simulink library "tpm"  (R2021b)
settings: Solver=VariableStepAuto  StartTime=0.0  StopTime=10.0  RelTol=1e-3
undefined symbols (not defined in the file or in its folder): ENUM_AN_LF, ENUM_AN_LR, ENUM_AN_RF, ENUM_AN_RR, ENUM_POWERSTA_OFF, ENUM_POWERSTA_OFFA, ENUM_POWERSTA_OFFC, ENUM_POWERSTA_ON, ENUM_POWERSTA_READY, ENUM_POWERSTA_STANDBY, ENUM_PWRSTASW_OFF, ENUM_PWRSTASW_OFFA, ENUM_PWRSTASW_OFFCHVCHRG, ENUM_PWRSTASW_STANDBY, ENUM_TPMSSNESORIDREGSTA_START, FALSE, KTPM_DataInVehSpdThreshold_kph, KTPM_Delay_raw8, KTPM_DiagLearn_flg, KTPM_TPMSModelVersion_raw, KTPM_TPMSModelVersionInit_raw, KTPM_WhlRotDir_enum_ovrdflg, KTPM_WhlRotDir_enum_ovrdval, TRUE, ZERO_FLOAT, ZERO_INT
libraries: simulink x58, $bdroot x27, hcu_lib x24
(part 6 of 9)

== system tpm/TPM/TPMS/TPMS/Learn/AutoLocation/IDIdentify/Subsystem3 ==
  VINP_DATAin_flg : Inport
  VINP_TPMSResButt_flg : Inport  Port=2
  VINP_IDin_raw32 : Inport  Port=3
  VTPM_LFWP_raw16 : Inport  Port=4
  VTPM_RFWP_raw16 : Inport  Port=5
  VTPM_LRWP_raw16 : Inport  Port=6
  VTPM_RRWP_raw16 : Inport  Port=7
  VPMM_PowerSta_enum : Inport  Port=8
  VINP_VehSpeed_kph : Inport  Port=9
  VINP_S4ID_raw : Inport  Port=10
  VTPM_TPMSmanualDone_flg : Inport  Port=11
  Add : Sum
  Chart : Stateflow chart  TreatAsAtomicUnit=on
      settings: PortSchema="{\"entries\":[{\"content\":{\"sides\":[{\"content\":{\"connectorIds\":[\"In1\",\"In2\",\"In3\",\"In5\",\"In7\",\"In4\",\"In6\"]},\"type\":\"ConnectorPlacement.EquallySpacedRectSide\",\"uuid\":\"84bbdee3-6a13-4113-bc08-a0b87ba22909\"},{\"content\":{\"connectorIds\":[\"Out5\",\"Out1\",\"Out4\",\"Out2\",\"Out3\"],\"side\":\"RIGHT\"},\"type\":\"ConnectorPlacement.EquallySpacedRectSide\",\"uuid\":\"b8796851-ab69-429f-9540-9571864c98e0\"},{\"content\":{\"connectorIds\":[],\"side\":\"TOP\"},\"type\":\"ConnectorPlacement.EquallySpacedRectSide\",\"uuid\":\"52bdbec4-409e-4a9a-a4bb-373a9525aed8\"}]},\"type\":\"ConnectorPlacement.EquallySpacedConnector\",\"uuid\":\"6e0a7370-38f8-4d4e-a3e7-eb2ef4c24b0f\"}],\"packageUris\":[\"http://schema.mathworks.com/mf0/Connector/R2020b\"],\"version\":\"1.0\"}"
  Chart1 : Stateflow chart  TreatAsAtomicUnit=on
      settings: PortSchema="{\"entries\":[{\"content\":{\"sides\":[{\"content\":{\"connectorIds\":[\"In2\",\"In1\",\"In3\",\"In4\",\"In5\",\"In6\",\"In7\",\"In8\"]},\"type\":\"ConnectorPlacement.EquallySpacedRectSide\",\"uuid\":\"0106c0c7-b0dd-4985-8477-027279f2cfbe\"},{\"content\":{\"connectorIds\":[\"Out1\",\"Out2\",\"Out3\",\"Out4\",\"Out5\"],\"side\":\"RIGHT\"},\"type\":\"ConnectorPlacement.EquallySpacedRectSide\",\"uuid\":\"38b36b5e-8790-43f5-89a8-de723ff40088\"},{\"content\":{\"connectorIds\":[],\"side\":\"TOP\"},\"type\":\"ConnectorPlacement.EquallySpacedRectSide\",\"uuid\":\"aa12a430-979d-4bba-b5af-88414204d80d\"}]},\"type\":\"ConnectorPlacement.EquallySpacedConnector\",\"uuid\":\"9f6249c4-6459-404e-8830-3ea500254943\"}],\"packageUris\":[\"http://schema.mathworks.com/mf0/Connector/R2020b\"],\"version\":\"1.0\"}"
  Constant : Constant  Value=ZERO_INT
  Constant18 : Constant  Value=0
  Constant5 : Constant  Value=KTPM_DataInVehSpdThreshold_kph  OutDataTypeStr=single
  Data Type Conversion10 : DataTypeConversion  OutDataTypeStr=uint32
  Detect Increase : simulink/Logic and Bit Operations/Detect Increase  vinit=0.0  OutDataTypeStr=boolean
  Enabled Subsystem1 : Subsystem  TreatAsAtomicUnit=on
  Enabled Subsystem2 : Subsystem  TreatAsAtomicUnit=on
  Enabled Subsystem3 : Subsystem  TreatAsAtomicUnit=on
  Enabled Subsystem5 : Subsystem  TreatAsAtomicUnit=on
  Logical Operator : Logic  Operator=OR  AllPortsSameDT=off  OutDataTypeStr=boolean
  NOT : Logic  Operator=NOT  IconShape=distinctive  AllPortsSameDT=off  OutDataTypeStr=boolean
  Relational Operator : RelationalOperator  Operator=~=  OutDataTypeStr=boolean  RndMeth=Simplest
  Switch5 : Switch  Criteria=u2 > Threshold
  Unit Delay1 : UnitDelay  SampleTime=-1  HasFrameUpgradeWarning=on
  IDOut : Outport
  VTPM_S4IDLock_flg : Outport  Port=2
  Used : Outport  Port=3
  VTPM_LFS4_cnt : Outport  Port=4
  VTPM_RFS4_cnt : Outport  Port=5
  VTPM_LRS4_cnt : Outport  Port=6
  VTPM_RRS4_cnt : Outport  Port=7
  C : Outport  Port=8
  GS4 : Outport  Port=9
  VTPM_S4timeout_flg : Outport  Port=10
  wires:
  VPMM_PowerSta_enum/1 -> Chart/2(VPMM_PowerSta_enum)
  Constant18/1 -> Switch5/1
  [VINP_TPMSResButt_flg] -> Switch5/2
  Data Type Conversion10/1 -> Add/1
  Unit Delay1/1 -> Add/2
  Switch5/1 -> [VTPM_GS4_cnt], Unit Delay1/1  "VTPM_GS4_cnt"
  Add/1 -> Switch5/3
  [C] -> Detect Increase/1
  Enabled Subsystem3/1(S) -> VTPM_RRS4_cnt/1
  Enabled Subsystem2/1(S) -> VTPM_LRS4_cnt/1
  Enabled Subsystem1/1(S) -> VTPM_RFS4_cnt/1
  [C] -> C/1
  Enabled Subsystem5/1(S) -> VTPM_LFS4_cnt/1
  Chart/3(RRM) -> Enabled Subsystem3/2(LFM1)
  [Cal] -> Enabled Subsystem3/Enable
  [C] -> Enabled Subsystem3/1(C)
  [C] -> Enabled Subsystem2/1(C)
  [Cal] -> Enabled Subsystem2/Enable
  Chart/2(LRM) -> Enabled Subsystem2/2(LFM1)
  Chart/4(RFM) -> Enabled Subsystem1/2(LFM1)
  [Cal] -> Enabled Subsystem1/Enable
  [C] -> Enabled Subsystem1/1(C)
  [C] -> Enabled Subsystem5/1(C)
  VINP_IDin_raw32/1 -> [VINP_IDin_raw32]
  VINP_TPMSResButt_flg/1 -> [VINP_TPMSResButt_flg]
  [VINP_TPMSResButt_flg] -> Logical Operator/2
  VTPM_RFWP_raw16/1 -> Chart/7(RF_PC)
  VTPM_RRWP_raw16/1 -> Chart/6(RR_PC)
  VTPM_LFWP_raw16/1 -> Chart/5(LF_PC)
  VTPM_LRWP_raw16/1 -> Chart/4(LR_PC)
  [G] -> Chart/3(GS)
  [VINP_TPMSResButt_flg] -> Chart1/2(VINP_TPMSResButt_flg)
  [VTPM_S4IDLock_flg] -> VTPM_S4IDLock_flg/1
  [VINP_IDin_raw32] -> Chart1/1(VINP_IDin_raw32)
  VINP_DATAin_flg/1 -> Chart1/3(VINP_DATAin_flg)
  Chart1/4(IDout) -> IDOut/1
  Chart1/1(G) -> GS4/1, [G], Data Type Conversion10/1
  Chart1/3(VTPM_S4IDLock_flg) -> [VTPM_S4IDLock_flg]
  Chart1/2(Used) -> [Used]
  [Used] -> Used/1
  Logical Operator/1 -> Chart/1(VINP_TPMSResButt_flg)
  [Used] -> NOT/1
  NOT/1 -> Logical Operator/1
  Chart/5(C) -> [C]
  [Cal] -> Enabled Subsystem5/Enable
  Chart/1(LFM) -> Enabled Subsystem5/2(LFM1)
  Detect Increase/1 -> [Cal]
  VINP_S4ID_raw/1 -> Relational Operator/1, [VINP_S4ID_raw]
  Constant/1 -> Relational Operator/2
  Relational Operator/1 -> [VTPM_FlashIDlock_flg]
  [VTPM_FlashIDlock_flg] -> Chart1/4(VTPM_FlashIDlock_flg)
  [VINP_S4ID_raw] -> Chart1/5(VINP_S4ID_raw)
  VINP_VehSpeed_kph/1 -> Chart1/6(VINP_VehSpeed_kph)
  Chart1/5(VTPM_S4timeout_flg) -> VTPM_S4timeout_flg/1
  VTPM_TPMSmanualDone_flg/1 -> Chart1/7(VTPM_TPMSmanualDone_flg)
  Constant5/1 -> Chart1/8(KTPM_DataInVehSpdThreshold_kph)

== system tpm/TPM/TPMS/TPMS/Learn/AutoLocation/IDIdentify/Subsystem7 ==
  VINP_DATAin_flg : Inport
  VINP_TPMSResButt_flg : Inport  Port=2
  VINP_IDin_raw32 : Inport  Port=3
  VTPM_LFWP_raw16 : Inport  Port=4
  VTPM_RFWP_raw16 : Inport  Port=5
  VTPM_LRWP_raw16 : Inport  Port=6
  VTPM_RRWP_raw16 : Inport  Port=7
  VPMM_PowerSta_enum : Inport  Port=8
  VINP_VehSpeed_kph : Inport  Port=9
  VINP_S1ID_raw : Inport  Port=10
  VTPM_TPMSmanualDone_flg : Inport  Port=11
  Add : Sum
  Chart : Stateflow chart  TreatAsAtomicUnit=on
      settings: PortSchema="{\"entries\":[{\"content\":{\"sides\":[{\"content\":{\"connectorIds\":[\"In1\",\"In2\",\"In3\",\"In5\",\"In7\",\"In4\",\"In6\"]},\"type\":\"ConnectorPlacement.EquallySpacedRectSide\",\"uuid\":\"84bbdee3-6a13-4113-bc08-a0b87ba22909\"},{\"content\":{\"connectorIds\":[\"Out5\",\"Out1\",\"Out4\",\"Out2\",\"Out3\"],\"side\":\"RIGHT\"},\"type\":\"ConnectorPlacement.EquallySpacedRectSide\",\"uuid\":\"b8796851-ab69-429f-9540-9571864c98e0\"},{\"content\":{\"connectorIds\":[],\"side\":\"TOP\"},\"type\":\"ConnectorPlacement.EquallySpacedRectSide\",\"uuid\":\"52bdbec4-409e-4a9a-a4bb-373a9525aed8\"}]},\"type\":\"ConnectorPlacement.EquallySpacedConnector\",\"uuid\":\"6e0a7370-38f8-4d4e-a3e7-eb2ef4c24b0f\"}],\"packageUris\":[\"http://schema.mathworks.com/mf0/Connector/R2020b\"],\"version\":\"1.0\"}"
  Chart1 : Stateflow chart  TreatAsAtomicUnit=on
      settings: PortSchema="{\"entries\":[{\"content\":{\"sides\":[{\"content\":{\"connectorIds\":[\"In2\",\"In1\",\"In3\",\"In4\",\"In5\",\"In6\",\"In7\",\"In8\"]},\"type\":\"ConnectorPlacement.EquallySpacedRectSide\",\"uuid\":\"0106c0c7-b0dd-4985-8477-027279f2cfbe\"},{\"content\":{\"connectorIds\":[\"Out1\",\"Out2\",\"Out3\",\"Out4\",\"Out5\"],\"side\":\"RIGHT\"},\"type\":\"ConnectorPlacement.EquallySpacedRectSide\",\"uuid\":\"38b36b5e-8790-43f5-89a8-de723ff40088\"},{\"content\":{\"connectorIds\":[],\"side\":\"TOP\"},\"type\":\"ConnectorPlacement.EquallySpacedRectSide\",\"uuid\":\"aa12a430-979d-4bba-b5af-88414204d80d\"}]},\"type\":\"ConnectorPlacement.EquallySpacedConnector\",\"uuid\":\"9f6249c4-6459-404e-8830-3ea500254943\"}],\"packageUris\":[\"http://schema.mathworks.com/mf0/Connector/R2020b\"],\"version\":\"1.0\"}"
  Constant : Constant  Value=ZERO_INT
  Constant18 : Constant  Value=0
  Constant5 : Constant  Value=KTPM_DataInVehSpdThreshold_kph  OutDataTypeStr=single
  Data Type Conversion10 : DataTypeConversion  OutDataTypeStr=uint32
  Detect Increase : simulink/Logic and Bit Operations/Detect Increase  vinit=0.0  OutDataTypeStr=boolean
  Enabled Subsystem1 : Subsystem  TreatAsAtomicUnit=on
  Enabled Subsystem2 : Subsystem  TreatAsAtomicUnit=on
  Enabled Subsystem3 : Subsystem  TreatAsAtomicUnit=on
  Enabled Subsystem5 : Subsystem  TreatAsAtomicUnit=on
  Logical Operator : Logic  Operator=OR  AllPortsSameDT=off  OutDataTypeStr=boolean
  NOT : Logic  Operator=NOT  IconShape=distinctive  AllPortsSameDT=off  OutDataTypeStr=boolean
  Relational Operator : RelationalOperator  Operator=~=  OutDataTypeStr=boolean  RndMeth=Simplest
  Switch5 : Switch  Criteria=u2 > Threshold
  Unit Delay1 : UnitDelay  SampleTime=-1  HasFrameUpgradeWarning=on
  IDOut : Outport
  VTPM_S1IDLock_flg : Outport  Port=2
  Used : Outport  Port=3
  VTPM_LFS1_cnt : Outport  Port=4
  VTPM_RFS1_cnt : Outport  Port=5
  VTPM_LRS1_cnt : Outport  Port=6
  VTPM_RRS1_cnt : Outport  Port=7
  C : Outport  Port=8
  GS1 : Outport  Port=9
  VTPM_S1timeout_flg : Outport  Port=10
  wires:
  Detect Increase/1 -> [Cal]
  Chart/1(LFM) -> Enabled Subsystem5/2(LFM1)
  [Cal] -> Enabled Subsystem5/Enable
  Chart/5(C) -> [C]
  NOT/1 -> Logical Operator/1
  [Used] -> NOT/1
  Logical Operator/1 -> Chart/1(VINP_TPMSResButt_flg)
  [Used] -> Used/1
  Chart1/2(Used) -> [Used]
  Chart1/3(VTPM_S1IDLock_flg) -> [VTPM_S1IDLock_flg]
  Chart1/1(G) -> Data Type Conversion10/1, GS1/1, [G]
  Chart1/4(IDout) -> IDOut/1
  VINP_DATAin_flg/1 -> Chart1/3(VINP_DATAin_flg)
  [VINP_IDin_raw32] -> Chart1/1(VINP_IDin_raw32)
  [VTPM_S1IDLock_flg] -> VTPM_S1IDLock_flg/1
  [VINP_TPMSResButt_flg] -> Chart1/2(VINP_TPMSResButt_flg)
  [G] -> Chart/3(GS)
  VTPM_LRWP_raw16/1 -> Chart/4(LR_PC)
  VTPM_LFWP_raw16/1 -> Chart/5(LF_PC)
  VTPM_RRWP_raw16/1 -> Chart/6(RR_PC)
  VTPM_RFWP_raw16/1 -> Chart/7(RF_PC)
  [VINP_TPMSResButt_flg] -> Logical Operator/2
  VINP_TPMSResButt_flg/1 -> [VINP_TPMSResButt_flg]
  VINP_IDin_raw32/1 -> [VINP_IDin_raw32]
  [C] -> Enabled Subsystem5/1(C)
  [C] -> Enabled Subsystem1/1(C)
  [Cal] -> Enabled Subsystem1/Enable
  Chart/4(RFM) -> Enabled Subsystem1/2(LFM1)
  Chart/2(LRM) -> Enabled Subsystem2/2(LFM1)
  [Cal] -> Enabled Subsystem2/Enable
  [C] -> Enabled Subsystem2/1(C)
  [C] -> Enabled Subsystem3/1(C)
  [Cal] -> Enabled Subsystem3/Enable
  Chart/3(RRM) -> Enabled Subsystem3/2(LFM1)
  Enabled Subsystem5/1(S) -> VTPM_LFS1_cnt/1
  [C] -> C/1
  Enabled Subsystem1/1(S) -> VTPM_RFS1_cnt/1
  Enabled Subsystem2/1(S) -> VTPM_LRS1_cnt/1
  Enabled Subsystem3/1(S) -> VTPM_RRS1_cnt/1
  [C] -> Detect Increase/1
  Add/1 -> Switch5/3
  Switch5/1 -> Unit Delay1/1, [VTPM_GS1_cnt]  "VTPM_GS1_cnt"
  Unit Delay1/1 -> Add/2
  Data Type Conversion10/1 -> Add/1
  [VINP_TPMSResButt_flg] -> Switch5/2
  Constant18/1 -> Switch5/1
  VPMM_PowerSta_enum/1 -> Chart/2(VPMM_PowerSta_enum)
  VINP_VehSpeed_kph/1 -> Chart1/6(VINP_VehSpeed_kph)
  VINP_S1ID_raw/1 -> [VINP_S1ID_raw], Relational Operator/1
  Relational Operator/1 -> [VTPM_FlashIDlock_flg]
  Constant/1 -> Relational Operator/2
  [VTPM_FlashIDlock_flg] -> Chart1/4(VTPM_FlashIDlock_flg)
  [VINP_S1ID_raw] -> Chart1/5(VINP_S1ID_raw)
  Chart1/5(VTPM_S1timeout_flg) -> VTPM_S1timeout_flg/1
  VTPM_TPMSmanualDone_flg/1 -> Chart1/7(VTPM_TPMSmanualDone_flg)
  Constant5/1 -> Chart1/8(KTPM_DataInVehSpdThreshold_kph)

== system tpm/TPM/TPMS/TPMS/Learn/AutoLocation/IDIdentify/unlearnsensorfail  ==
  VTPM_ALLFIN_flg : Inport
  VINP_VehSpeed_kph : Inport  Port=2
  VTPM_IDLOCK_flg : Inport  Port=3
  GS1 : Inport  Port=4
  GS2 : Inport  Port=5
  GS3 : Inport  Port=6
  GS4 : Inport  Port=7
  VINP_TPMSResButt_flg : Inport  Port=8
  VINP_FlashunlearnSfali_flg : Inport  Port=9
  VINP_ChkStorge_flg : Inport  Port=10
  VINP_TPMSStorge_flg : Inport  Port=11
  VTPM_TPMSmanualDone_flg : Inport  Port=12
  Chart : Stateflow chart  TreatAsAtomicUnit=on
      settings: PortSchema="{\"entries\":[{\"content\":{\"sides\":[{\"content\":{\"connectorIds\":[\"In1\",\"In2\",\"In3\",\"In7\",\"In4\",\"In5\",\"In6\",\"In8\",\"In9\",\"In10\",\"In11\",\"In12\"]},\"type\":\"ConnectorPlacement.EquallySpacedRectSide\",\"uuid\":\"6d6ad79b-53cb-4fcc-b2ed-afc1b708014e\"},{\"content\":{\"connectorIds\":[\"Out1\",\"Out2\"],\"side\":\"RIGHT\"},\"type\":\"ConnectorPlacement.EquallySpacedRectSide\",\"uuid\":\"e1142f2b-ba58-4cb3-ba57-f7dfdeb40e8a\"},{\"content\":{\"connectorIds\":[],\"side\":\"TOP\"},\"type\":\"ConnectorPlacement.EquallySpacedRectSide\",\"uuid\":\"d6c2cba7-0cc1-4e16-8027-e1abdfd1a8ea\"}]},\"type\":\"ConnectorPlacement.EquallySpacedConnector\",\"uuid\":\"635c654b-7cdc-40ae-8580-2307d04d13e7\"}],\"packageUris\":[\"http://schema.mathworks.com/mf0/Connector/R2020b\"],\"version\":\"1.0\"}"
  Detect Increase4 : simulink/Logic and Bit Operations/Detect Increase  vinit=0.0  OutDataTypeStr=boolean
  SR_Latch : hcu_lib/Basic_Blocks/SR_Latch
  SR_Latch1 : hcu_lib/Basic_Blocks/SR_Latch
  VTPM_unlearnSfali_flg : Outport
  VTPM_unlearnSfailvalid_enum : Outport  Port=2
  VTPM_unlockpopup_flg : Outport  Port=3
  wires:
  Chart/1(VTPM_unlearnSfali_flg) -> VTPM_unlearnSfali_flg/1, [VTPM_unlearnSfali_flg]
  GS1/1 -> Chart/7(VTPM_GS1_flg)
  GS4/1 -> Chart/6(VTPM_GS4_flg)
  GS3/1 -> Chart/5(VTPM_GS3_flg)
  GS2/1 -> Chart/4(VTPM_GS2_flg)
  VTPM_IDLOCK_flg/1 -> Chart/3(VTPM_IDLOCK_flg)
  VINP_VehSpeed_kph/1 -> Chart/2(VINP_VehSpeed_kph)
  VTPM_ALLFIN_flg/1 -> Chart/1(VTPM_ALLFIN_flg)
  VINP_FlashunlearnSfali_flg/1 -> Chart/9(VINP_FlashunlearnSfali_flg)
  VINP_ChkStorge_flg/1 -> Chart/10(VINP_ChkStorge_flg)
  VINP_TPMSStorge_flg/1 -> Chart/11(VINP_TPMSStorge_flg)
  SR_Latch/1 -> VTPM_unlearnSfailvalid_enum/1
  Detect Increase4/1 -> SR_Latch/1
  [VTPM_unlearnSfali_flg] -> Detect Increase4/1
  VINP_TPMSResButt_flg/1 -> [VINP_TPMSResButt_flg]
  [VINP_TPMSResButt_flg] -> Chart/8(VINP_TPMSResButt_flg)
  [VINP_TPMSResButt_flg] -> SR_Latch/2
  Chart/2(VTPM_unlockpopup_flg) -> VTPM_unlockpopup_flg/1
  VTPM_TPMSmanualDone_flg/1 -> SR_Latch1/1
  SR_Latch1/1 -> Chart/12(VTPM_TPMSmanualDone_flg)
  [VINP_TPMSResButt_flg] -> SR_Latch1/2

== system tpm/TPM/TPMS/TPMS/Learn/AutoLocation/Subsystem1/Subsystem ==
  VTPM_ManualID1_raw : Inport
  VTPM_ManualID2_raw : Inport  Port=2
  VTPM_ManualID3_raw : Inport  Port=3
  VTPM_ManualID4_raw : Inport  Port=4
  VTPM_TPMSmanualDone_flg : Inport  Port=5
  VINP_TPMSResButt_flg : Inport  Port=6
  VINP_LFID_raw : Inport  Port=7
  VINP_RFID_raw : Inport  Port=8
  VINP_LRID_raw : Inport  Port=9
  VINP_RRID_raw : Inport  Port=10
  VINP_S1ID_raw : Inport  Port=11
  VINP_S2ID_raw : Inport  Port=12
  VINP_S3ID_raw : Inport  Port=13
  VINP_S4ID_raw : Inport  Port=14
  VINP_TPMSStorge_flg : Inport  Port=15
  Chart : Stateflow chart  TreatAsAtomicUnit=on
  VTPM_MSensor1ID_raw : Outport
  VTPM_MSensor2ID_raw : Outport  Port=2
  VTPM_MSensor3ID_raw : Outport  Port=3
  VTPM_MSensor4ID_raw : Outport  Port=4
  VTPM_TPMSStorge_flg : Outport  Port=5
  VTPM_MLFID_raw : Outport  Port=6
  VTPM_MLRID_raw : Outport  Port=7
  VTPM_MRFID_raw : Outport  Port=8
  VTPM_MRRID_raw : Outport  Port=9
  wires:
  VTPM_ManualID1_raw/1 -> Chart/7(VTPM_ManualID1_raw)
  VTPM_ManualID2_raw/1 -> Chart/8(VTPM_ManualID2_raw)
  VTPM_ManualID3_raw/1 -> Chart/9(VTPM_ManualID3_raw)
  VTPM_ManualID4_raw/1 -> Chart/10(VTPM_ManualID4_raw)
  Chart/1(VTPM_MSensor1ID_raw) -> VTPM_MSensor1ID_raw/1
  Chart/2(VTPM_MSensor2ID_raw) -> VTPM_MSensor2ID_raw/1
  Chart/3(VTPM_MSensor3ID_raw) -> VTPM_MSensor3ID_raw/1
  Chart/4(VTPM_MSensor4ID_raw) -> VTPM_MSensor4ID_raw/1
  VTPM_TPMSmanualDone_flg/1 -> Chart/1(VTPM_TPMSmanualDone_flg)
  VINP_TPMSResButt_flg/1 -> Chart/2(VINP_TPMSResButt_flg)
  Chart/5(VTPM_TPMSStorge_flg) -> VTPM_TPMSStorge_flg/1
  VINP_RRID_raw/1 -> Chart/6(VINP_RRID_raw)
  VINP_LRID_raw/1 -> Chart/5(VINP_LRID_raw)
  VINP_RFID_raw/1 -> Chart/4(VINP_RFID_raw)
  VINP_LFID_raw/1 -> Chart/3(VINP_LFID_raw)
  VINP_S1ID_raw/1 -> Chart/11(VINP_S1ID_raw)
  VINP_S2ID_raw/1 -> Chart/12(VINP_S2ID_raw)
  VINP_S3ID_raw/1 -> Chart/13(VINP_S3ID_raw)
  VINP_S4ID_raw/1 -> Chart/14(VINP_S4ID_raw)
  Chart/6(VTPM_MLFID_raw) -> VTPM_MLFID_raw/1
  Chart/7(VTPM_MLRID_raw) -> VTPM_MLRID_raw/1
  Chart/8(VTPM_MRFID_raw) -> VTPM_MRFID_raw/1
  Chart/9(VTPM_MRRID_raw) -> VTPM_MRRID_raw/1
  VINP_TPMSStorge_flg/1 -> Chart/15(VINP_TPMSStorge_flg)

== system tpm/TPM/TPMS/TPMS/Learn/AutoLocation/WheelPosition/Subsystem ==
  VTPM_LFWpos_raw : Inport
  Constant : Constant  Value=KTPM_Delay_raw8
  If : If  IfExpression=u1 == 1  ElseIfExpressions=u1 ==2,u1 ==3,u1 ==4,u1 == 5,u1 ==6,u1 ==7,u1 ==8
  Merge1 : Merge  Inputs=9
  delay0 : Subsystem  TreatAsAtomicUnit=on
  delay1 : Subsystem  TreatAsAtomicUnit=on
  delay2 : Subsystem  TreatAsAtomicUnit=on
  delay3 : Subsystem  TreatAsAtomicUnit=on
  delay4 : Subsystem  TreatAsAtomicUnit=on
  delay5 : Subsystem  TreatAsAtomicUnit=on
  delay6 : Subsystem  TreatAsAtomicUnit=on
  delay7 : Subsystem  TreatAsAtomicUnit=on
  delay8 : Subsystem  TreatAsAtomicUnit=on
  VTPM_LFWP_raw16 : Outport
  wires:
  [VTPM_LFWP_raw16] -> delay3/1(In1)
  [VTPM_LFWP_raw16] -> delay1/1(In1)
  Constant/1 -> If/1
  Merge1/1 -> VTPM_LFWP_raw16/1
  [VTPM_LFWP_raw16] -> delay6/1(In1)
  [VTPM_LFWP_raw16] -> delay5/1(In1)
  [VTPM_LFWP_raw16] -> delay2/1(In1)
  [VTPM_LFWP_raw16] -> delay4/1(In1)
  [VTPM_LFWP_raw16] -> delay0/1(In1)
  VTPM_LFWpos_raw/1 -> [VTPM_LFWP_raw16]
  If/1 -> delay1/Action
  If/2 -> delay2/Action
  If/3 -> delay3/Action
  If/4 -> delay4/Action
  If/5 -> delay5/Action
  If/6 -> delay6/Action
  If/9 -> delay0/Action
  delay5/1(Out1) -> Merge1/5
  delay4/1(Out1) -> Merge1/4
  delay1/1(Out1) -> Merge1/1
  delay3/1(Out1) -> Merge1/3
  delay6/1(Out1) -> Merge1/6
  delay2/1(Out1) -> Merge1/2
  If/7 -> delay7/Action
  [VTPM_LFWP_raw16] -> delay7/1(In1)
  [VTPM_LFWP_raw16] -> delay8/1(In1)
  If/8 -> delay8/Action
  delay7/1(Out1) -> Merge1/7
  delay8/1(Out1) -> Merge1/8
  delay0/1(Out1) -> Merge1/9

== system tpm/TPM/TPMS/TPMS/Learn/AutoLocation/WheelPosition/Subsystem1 ==
  VTPM_RFWpos_raw : Inport
  Constant : Constant  Value=KTPM_Delay_raw8
  If : If  IfExpression=u1 == 1  ElseIfExpressions=u1 ==2,u1 ==3,u1 ==4,u1 == 5,u1 ==6,u1 ==7,u1 ==8
  Merge1 : Merge  Inputs=9
  delay0 : $bdroot/TPM/TPMS/TPMS/Learn/AutoLocation/WheelPosition/Subsystem/delay0  SystemSampleTime=-1  VariantActivationTime=update diagram  Latency=0  AutoFrameSizeCalculation=off
  delay1 : $bdroot/TPM/TPMS/TPMS/Learn/AutoLocation/WheelPosition/Subsystem/delay1  SystemSampleTime=-1  VariantActivationTime=update diagram  Latency=0  AutoFrameSizeCalculation=off
  delay2 : $bdroot/TPM/TPMS/TPMS/Learn/AutoLocation/WheelPosition/Subsystem/delay2  SystemSampleTime=-1  VariantActivationTime=update diagram  Latency=0  AutoFrameSizeCalculation=off
  delay3 : $bdroot/TPM/TPMS/TPMS/Learn/AutoLocation/WheelPosition/Subsystem/delay3  SystemSampleTime=-1  VariantActivationTime=update diagram  Latency=0  AutoFrameSizeCalculation=off
  delay4 : $bdroot/TPM/TPMS/TPMS/Learn/AutoLocation/WheelPosition/Subsystem/delay4  SystemSampleTime=-1  VariantActivationTime=update diagram  Latency=0  AutoFrameSizeCalculation=off
  delay5 : $bdroot/TPM/TPMS/TPMS/Learn/AutoLocation/WheelPosition/Subsystem/delay5  SystemSampleTime=-1  VariantActivationTime=update diagram  Latency=0  AutoFrameSizeCalculation=off
  delay6 : $bdroot/TPM/TPMS/TPMS/Learn/AutoLocation/WheelPosition/Subsystem/delay6  SystemSampleTime=-1  VariantActivationTime=update diagram  Latency=0  AutoFrameSizeCalculation=off
  delay7 : $bdroot/TPM/TPMS/TPMS/Learn/AutoLocation/WheelPosition/Subsystem/delay7  SystemSampleTime=-1  VariantActivationTime=update diagram  Latency=0  AutoFrameSizeCalculation=off
  delay8 : $bdroot/TPM/TPMS/TPMS/Learn/AutoLocation/WheelPosition/Subsystem/delay8  SystemSampleTime=-1  VariantActivationTime=update diagram  Latency=0  AutoFrameSizeCalculation=off
  VTPM_RFWP_raw16 : Outport
  wires:
  Merge1/1 -> VTPM_RFWP_raw16/1
  VTPM_RFWpos_raw/1 -> [VTPM_RFWP_raw16]
  [VTPM_RFWP_raw16] -> delay7/1
  delay7/1 -> Merge1/7
  delay8/1 -> Merge1/8
  delay0/1 -> Merge1/9
  [VTPM_RFWP_raw16] -> delay8/1
  [VTPM_RFWP_raw16] -> delay3/1
  If/2 -> delay2/Action
  [VTPM_RFWP_raw16] -> delay2/1
  [VTPM_RFWP_raw16] -> delay4/1
  If/1 -> delay1/Action
  [VTPM_RFWP_raw16] -> delay1/1
  If/9 -> delay0/Action
  If/3 -> delay3/Action
  [VTPM_RFWP_raw16] -> delay0/1
  delay2/1 -> Merge1/2
  delay5/1 -> Merge1/5
  [VTPM_RFWP_raw16] -> delay5/1
  delay6/1 -> Merge1/6
  If/6 -> delay6/Action
  If/8 -> delay8/Action
  delay3/1 -> Merge1/3
  If/5 -> delay5/Action
  [VTPM_RFWP_raw16] -> delay6/1
  If/4 -> delay4/Action
  delay4/1 -> Merge1/4
  delay1/1 -> Merge1/1
  If/7 -> delay7/Action
  Constant/1 -> If/1

== system tpm/TPM/TPMS/TPMS/Learn/AutoLocation/WheelPosition/Subsystem2 ==
  VTPM_LRWpos_raw : Inport
  Constant : Constant  Value=KTPM_Delay_raw8
  If : If  IfExpression=u1 == 1  ElseIfExpressions=u1 ==2,u1 ==3,u1 ==4,u1 == 5,u1 ==6,u1 ==7,u1 ==8
  Merge1 : Merge  Inputs=9
  delay0 : $bdroot/TPM/TPMS/TPMS/Learn/AutoLocation/WheelPosition/Subsystem/delay0  SystemSampleTime=-1  VariantActivationTime=update diagram  Latency=0  AutoFrameSizeCalculation=off
  delay1 : $bdroot/TPM/TPMS/TPMS/Learn/AutoLocation/WheelPosition/Subsystem/delay1  SystemSampleTime=-1  VariantActivationTime=update diagram  Latency=0  AutoFrameSizeCalculation=off
  delay2 : $bdroot/TPM/TPMS/TPMS/Learn/AutoLocation/WheelPosition/Subsystem/delay2  SystemSampleTime=-1  VariantActivationTime=update diagram  Latency=0  AutoFrameSizeCalculation=off
  delay3 : $bdroot/TPM/TPMS/TPMS/Learn/AutoLocation/WheelPosition/Subsystem/delay3  SystemSampleTime=-1  VariantActivationTime=update diagram  Latency=0  AutoFrameSizeCalculation=off
  delay4 : $bdroot/TPM/TPMS/TPMS/Learn/AutoLocation/WheelPosition/Subsystem/delay4  SystemSampleTime=-1  VariantActivationTime=update diagram  Latency=0  AutoFrameSizeCalculation=off
  delay5 : $bdroot/TPM/TPMS/TPMS/Learn/AutoLocation/WheelPosition/Subsystem/delay5  SystemSampleTime=-1  VariantActivationTime=update diagram  Latency=0  AutoFrameSizeCalculation=off
  delay6 : $bdroot/TPM/TPMS/TPMS/Learn/AutoLocation/WheelPosition/Subsystem/delay6  SystemSampleTime=-1  VariantActivationTime=update diagram  Latency=0  AutoFrameSizeCalculation=off
  delay7 : $bdroot/TPM/TPMS/TPMS/Learn/AutoLocation/WheelPosition/Subsystem/delay7  SystemSampleTime=-1  VariantActivationTime=update diagram  Latency=0  AutoFrameSizeCalculation=off
  delay8 : $bdroot/TPM/TPMS/TPMS/Learn/AutoLocation/WheelPosition/Subsystem/delay8  SystemSampleTime=-1  VariantActivationTime=update diagram  Latency=0  AutoFrameSizeCalculation=off
  VTPM_LRWP_raw16 : Outport
  wires:
  VTPM_LRWpos_raw/1 -> [VTPM_LRWP_raw16]
  Constant/1 -> If/1
  [VTPM_LRWP_raw16] -> delay5/1
  delay6/1 -> Merge1/6
  If/7 -> delay7/Action
  delay1/1 -> Merge1/1
  delay4/1 -> Merge1/4
  If/4 -> delay4/Action
  If/5 -> delay5/Action
  delay3/1 -> Merge1/3
  delay5/1 -> Merge1/5
  If/6 -> delay6/Action
  [VTPM_LRWP_raw16] -> delay0/1
  If/3 -> delay3/Action
  [VTPM_LRWP_raw16] -> delay3/1
  If/9 -> delay0/Action
  [VTPM_LRWP_raw16] -> delay8/1
  [VTPM_LRWP_raw16] -> delay2/1
  If/2 -> delay2/Action
  If/1 -> delay1/Action
  [VTPM_LRWP_raw16] -> delay1/1
  [VTPM_LRWP_raw16] -> delay4/1
  delay2/1 -> Merge1/2
  delay0/1 -> Merge1/9
  [VTPM_LRWP_raw16] -> delay7/1
  delay7/1 -> Merge1/7
  If/8 -> delay8/Action
  delay8/1 -> Merge1/8
  [VTPM_LRWP_raw16] -> delay6/1
  Merge1/1 -> VTPM_LRWP_raw16/1

== system tpm/TPM/TPMS/TPMS/Learn/AutoLocation/WheelPosition/Subsystem3 ==
  VTPM_RRWpos_raw : Inport
  Constant : Constant  Value=KTPM_Delay_raw8
  If : If  IfExpression=u1 == 1  ElseIfExpressions=u1 ==2,u1 ==3,u1 ==4,u1 == 5,u1 ==6,u1 ==7,u1 ==8
  Merge1 : Merge  Inputs=9
  delay0 : $bdroot/TPM/TPMS/TPMS/Learn/AutoLocation/WheelPosition/Subsystem/delay0  SystemSampleTime=-1  VariantActivationTime=update diagram  Latency=0  AutoFrameSizeCalculation=off
  delay1 : $bdroot/TPM/TPMS/TPMS/Learn/AutoLocation/WheelPosition/Subsystem/delay1  SystemSampleTime=-1  VariantActivationTime=update diagram  Latency=0  AutoFrameSizeCalculation=off
  delay2 : $bdroot/TPM/TPMS/TPMS/Learn/AutoLocation/WheelPosition/Subsystem/delay2  SystemSampleTime=-1  VariantActivationTime=update diagram  Latency=0  AutoFrameSizeCalculation=off
  delay3 : $bdroot/TPM/TPMS/TPMS/Learn/AutoLocation/WheelPosition/Subsystem/delay3  SystemSampleTime=-1  VariantActivationTime=update diagram  Latency=0  AutoFrameSizeCalculation=off
  delay4 : $bdroot/TPM/TPMS/TPMS/Learn/AutoLocation/WheelPosition/Subsystem/delay4  SystemSampleTime=-1  VariantActivationTime=update diagram  Latency=0  AutoFrameSizeCalculation=off
  delay5 : $bdroot/TPM/TPMS/TPMS/Learn/AutoLocation/WheelPosition/Subsystem/delay5  SystemSampleTime=-1  VariantActivationTime=update diagram  Latency=0  AutoFrameSizeCalculation=off
  delay6 : $bdroot/TPM/TPMS/TPMS/Learn/AutoLocation/WheelPosition/Subsystem/delay6  SystemSampleTime=-1  VariantActivationTime=update diagram  Latency=0  AutoFrameSizeCalculation=off
  delay7 : $bdroot/TPM/TPMS/TPMS/Learn/AutoLocation/WheelPosition/Subsystem/delay7  SystemSampleTime=-1  VariantActivationTime=update diagram  Latency=0  AutoFrameSizeCalculation=off
  delay8 : $bdroot/TPM/TPMS/TPMS/Learn/AutoLocation/WheelPosition/Subsystem/delay8  SystemSampleTime=-1  VariantActivationTime=update diagram  Latency=0  AutoFrameSizeCalculation=off
  VTPM_RRWP_raw16 : Outport
  wires:
  Merge1/1 -> VTPM_RRWP_raw16/1
  [VTPM_RRWP_raw16] -> delay6/1
  delay8/1 -> Merge1/8
  If/8 -> delay8/Action
  delay7/1 -> Merge1/7
  [VTPM_RRWP_raw16] -> delay7/1
  delay0/1 -> Merge1/9
  delay2/1 -> Merge1/2
  [VTPM_RRWP_raw16] -> delay4/1
  [VTPM_RRWP_raw16] -> delay1/1
  If/1 -> delay1/Action
  If/2 -> delay2/Action
  [VTPM_RRWP_raw16] -> delay2/1
  [VTPM_RRWP_raw16] -> delay8/1
  If/9 -> delay0/Action
  [VTPM_RRWP_raw16] -> delay3/1
  If/3 -> delay3/Action
  [VTPM_RRWP_raw16] -> delay0/1
  If/6 -> delay6/Action
  delay5/1 -> Merge1/5
  delay3/1 -> Merge1/3
  If/5 -> delay5/Action
  If/4 -> delay4/Action
  delay4/1 -> Merge1/4
  delay1/1 -> Merge1/1
  If/7 -> delay7/Action
  delay6/1 -> Merge1/6
  [VTPM_RRWP_raw16] -> delay5/1
  Constant/1 -> If/1
  VTPM_RRWpos_raw/1 -> [VTPM_RRWP_raw16]

== system tpm/TPM/TPMS/TPMS/Learn/AutoLocation/IDIdentify/Subsystem1/Enabled Subsystem1 ==
  C : Inport
  LFM1 : Inport  Port=2
  Enable : EnablePort
  Data Type Conversion{1..8} (8 alike) : DataTypeConversion  OutDataTypeStr=int16
  Data Type Conversion9 : DataTypeConversion  OutDataTypeStr=uint8
  MATLAB Function : MATLAB Function  TreatAsAtomicUnit=on
  Unit Delay{1..8} (8 alike) : UnitDelay  SampleTime=-1  HasFrameUpgradeWarning=on
  S : Outport
  wires:
  Data Type Conversion9/1 -> S/1
  Data Type Conversion3/1 -> [X4]
  Data Type Conversion2/1 -> [X3]
  Data Type Conversion1/1 -> [X2]
  LFM1/1 -> MATLAB Function/2(Min)
  MATLAB Function/1(S) -> Data Type Conversion9/1
  C/1 -> MATLAB Function/1(C)
  MATLAB Function/2(Y2) -> Unit Delay1/1
  MATLAB Function/3(Y3) -> Unit Delay2/1
  MATLAB Function/4(Y4) -> Unit Delay3/1
  Unit Delay1/1 -> Data Type Conversion1/1
  Unit Delay2/1 -> Data Type Conversion2/1
  Unit Delay3/1 -> Data Type Conversion3/1
  [X2] -> MATLAB Function/3(X2)
  [X3] -> MATLAB Function/4(X3)
  [X4] -> MATLAB Function/5(X4)
  Unit Delay6/1 -> Data Type Conversion5/1
  Unit Delay5/1 -> Data Type Conversion4/1
  MATLAB Function/6(Y6) -> Unit Delay6/1
  MATLAB Function/5(Y5) -> Unit Delay5/1
  Data Type Conversion4/1 -> [X5]
  Data Type Conversion5/1 -> [X6]
  [X5] -> MATLAB Function/6(X5)
  [X6] -> MATLAB Function/7(X6)
  [X7] -> MATLAB Function/8(X7)
  [X8] -> MATLAB Function/9(X8)
  Data Type Conversion6/1 -> [X7]
  MATLAB Function/7(Y7) -> Unit Delay4/1
  Unit Delay4/1 -> Data Type Conversion6/1
  Unit Delay7/1 -> Data Type Conversion7/1
  Data Type Conversion7/1 -> [X8]
  MATLAB Function/8(Y8) -> Unit Delay7/1
  MATLAB Function/9(Y9) -> Unit Delay8/1
  Data Type Conversion8/1 -> [X9]
  Unit Delay8/1 -> Data Type Conversion8/1
  [X9] -> MATLAB Function/10(X9)

== system tpm/TPM/TPMS/TPMS/Learn/AutoLocation/IDIdentify/Subsystem1/Enabled Subsystem2 ==
  C : Inport
  LFM1 : Inport  Port=2
  Enable : EnablePort
  Data Type Conversion{1..8} (8 alike) : DataTypeConversion  OutDataTypeStr=int16
  Data Type Conversion9 : DataTypeConversion  OutDataTypeStr=uint8
  MATLAB Function : MATLAB Function  TreatAsAtomicUnit=on
  Unit Delay{1..8} (8 alike) : UnitDelay  SampleTime=-1  HasFrameUpgradeWarning=on
  S : Outport
  wires:
  Data Type Conversion9/1 -> S/1
  [X9] -> MATLAB Function/10(X9)
  Unit Delay8/1 -> Data Type Conversion8/1
  Data Type Conversion8/1 -> [X9]
  MATLAB Function/9(Y9) -> Unit Delay8/1
  MATLAB Function/8(Y8) -> Unit Delay7/1
  Data Type Conversion7/1 -> [X8]
  Unit Delay7/1 -> Data Type Conversion7/1
  Unit Delay4/1 -> Data Type Conversion6/1
  MATLAB Function/7(Y7) -> Unit Delay4/1
  Data Type Conversion6/1 -> [X7]
  [X8] -> MATLAB Function/9(X8)
  [X7] -> MATLAB Function/8(X7)
  [X6] -> MATLAB Function/7(X6)
  [X5] -> MATLAB Function/6(X5)
  Data Type Conversion5/1 -> [X6]
  Data Type Conversion4/1 -> [X5]
  MATLAB Function/5(Y5) -> Unit Delay5/1
  MATLAB Function/6(Y6) -> Unit Delay6/1
  Unit Delay5/1 -> Data Type Conversion4/1
  Unit Delay6/1 -> Data Type Conversion5/1
  [X4] -> MATLAB Function/5(X4)
  [X3] -> MATLAB Function/4(X3)
  [X2] -> MATLAB Function/3(X2)
  Unit Delay3/1 -> Data Type Conversion3/1
  Unit Delay2/1 -> Data Type Conversion2/1
  Unit Delay1/1 -> Data Type Conversion1/1
  MATLAB Function/4(Y4) -> Unit Delay3/1
  MATLAB Function/3(Y3) -> Unit Delay2/1
  MATLAB Function/2(Y2) -> Unit Delay1/1
  C/1 -> MATLAB Function/1(C)
  MATLAB Function/1(S) -> Data Type Conversion9/1
  LFM1/1 -> MATLAB Function/2(Min)
  Data Type Conversion1/1 -> [X2]
  Data Type Conversion2/1 -> [X3]
  Data Type Conversion3/1 -> [X4]

== system tpm/TPM/TPMS/TPMS/Learn/AutoLocation/IDIdentify/Subsystem1/Enabled Subsystem3 ==
  C : Inport
  LFM1 : Inport  Port=2
  Enable : EnablePort
  Data Type Conversion{1..8} (8 alike) : DataTypeConversion  OutDataTypeStr=int16
  Data Type Conversion9 : DataTypeConversion  OutDataTypeStr=uint8
  MATLAB Function : MATLAB Function  TreatAsAtomicUnit=on
  Unit Delay{1..8} (8 alike) : UnitDelay  SampleTime=-1  HasFrameUpgradeWarning=on
  S : Outport
  wires:
  Data Type Conversion9/1 -> S/1
  Data Type Conversion3/1 -> [X4]
  Data Type Conversion2/1 -> [X3]
  Data Type Conversion1/1 -> [X2]
  LFM1/1 -> MATLAB Function/2(Min)
  MATLAB Function/1(S) -> Data Type Conversion9/1
  C/1 -> MATLAB Function/1(C)
  MATLAB Function/2(Y2) -> Unit Delay1/1
  MATLAB Function/3(Y3) -> Unit Delay2/1
  MATLAB Function/4(Y4) -> Unit Delay3/1
  Unit Delay1/1 -> Data Type Conversion1/1
  Unit Delay2/1 -> Data Type Conversion2/1
  Unit Delay3/1 -> Data Type Conversion3/1
  [X2] -> MATLAB Function/3(X2)
  [X3] -> MATLAB Function/4(X3)
  [X4] -> MATLAB Function/5(X4)
  Unit Delay6/1 -> Data Type Conversion5/1
  Unit Delay5/1 -> Data Type Conversion4/1
  MATLAB Function/6(Y6) -> Unit Delay6/1
  MATLAB Function/5(Y5) -> Unit Delay5/1
  Data Type Conversion4/1 -> [X5]
  Data Type Conversion5/1 -> [X6]
  [X5] -> MATLAB Function/6(X5)
  [X6] -> MATLAB Function/7(X6)
  [X7] -> MATLAB Function/8(X7)
  [X8] -> MATLAB Function/9(X8)
  Data Type Conversion6/1 -> [X7]
  MATLAB Function/7(Y7) -> Unit Delay4/1
  Unit Delay4/1 -> Data Type Conversion6/1
  Unit Delay7/1 -> Data Type Conversion7/1
  Data Type Conversion7/1 -> [X8]
  MATLAB Function/8(Y8) -> Unit Delay7/1
  MATLAB Function/9(Y9) -> Unit Delay8/1
  Data Type Conversion8/1 -> [X9]
  Unit Delay8/1 -> Data Type Conversion8/1
  [X9] -> MATLAB Function/10(X9)

== system tpm/TPM/TPMS/TPMS/Learn/AutoLocation/IDIdentify/Subsystem1/Enabled Subsystem5 ==
  C : Inport
  LFM1 : Inport  Port=2
  Enable : EnablePort
  Data Type Conversion{1..8} (8 alike) : DataTypeConversion  OutDataTypeStr=int16
  Data Type Conversion9 : DataTypeConversion  OutDataTypeStr=uint8
  MATLAB Function : MATLAB Function  TreatAsAtomicUnit=on
  Unit Delay{1..8} (8 alike) : UnitDelay  SampleTime=-1  HasFrameUpgradeWarning=on
  S : Outport
  wires:
  Data Type Conversion9/1 -> S/1
  [X9] -> MATLAB Function/10(X9)
  Unit Delay8/1 -> Data Type Conversion8/1
  Data Type Conversion8/1 -> [X9]
  MATLAB Function/9(Y9) -> Unit Delay8/1
  MATLAB Function/8(Y8) -> Unit Delay7/1
  Data Type Conversion7/1 -> [X8]
  Unit Delay7/1 -> Data Type Conversion7/1
  Unit Delay4/1 -> Data Type Conversion6/1
  MATLAB Function/7(Y7) -> Unit Delay4/1
  Data Type Conversion6/1 -> [X7]
  [X8] -> MATLAB Function/9(X8)
  [X7] -> MATLAB Function/8(X7)
  [X6] -> MATLAB Function/7(X6)
  [X5] -> MATLAB Function/6(X5)
  Data Type Conversion5/1 -> [X6]
  Data Type Conversion4/1 -> [X5]
  MATLAB Function/5(Y5) -> Unit Delay5/1
  MATLAB Function/6(Y6) -> Unit Delay6/1
  Unit Delay5/1 -> Data Type Conversion4/1
  Unit Delay6/1 -> Data Type Conversion5/1
  [X4] -> MATLAB Function/5(X4)
  [X3] -> MATLAB Function/4(X3)
  [X2] -> MATLAB Function/3(X2)
  Unit Delay3/1 -> Data Type Conversion3/1
  Unit Delay2/1 -> Data Type Conversion2/1
  Unit Delay1/1 -> Data Type Conversion1/1
  MATLAB Function/4(Y4) -> Unit Delay3/1
  MATLAB Function/3(Y3) -> Unit Delay2/1
  MATLAB Function/2(Y2) -> Unit Delay1/1
  C/1 -> MATLAB Function/1(C)
  MATLAB Function/1(S) -> Data Type Conversion9/1
  LFM1/1 -> MATLAB Function/2(Min)
  Data Type Conversion1/1 -> [X2]
  Data Type Conversion2/1 -> [X3]
  Data Type Conversion3/1 -> [X4]

== system tpm/TPM/TPMS/TPMS/Learn/AutoLocation/IDIdentify/Subsystem2/Enabled Subsystem1 ==
  C : Inport
  LFM1 : Inport  Port=2
  Enable : EnablePort
  Data Type Conversion{1..8} (8 alike) : DataTypeConversion  OutDataTypeStr=int16
  Data Type Conversion9 : DataTypeConversion  OutDataTypeStr=uint8
  MATLAB Function : MATLAB Function  TreatAsAtomicUnit=on
  Unit Delay{1..8} (8 alike) : UnitDelay  SampleTime=-1  HasFrameUpgradeWarning=on
  S : Outport
  wires:
  [X9] -> MATLAB Function/10(X9)
  Unit Delay8/1 -> Data Type Conversion8/1
  Data Type Conversion8/1 -> [X9]
  MATLAB Function/9(Y9) -> Unit Delay8/1
  MATLAB Function/8(Y8) -> Unit Delay7/1
  Data Type Conversion7/1 -> [X8]
  Unit Delay7/1 -> Data Type Conversion7/1
  Unit Delay4/1 -> Data Type Conversion6/1
  MATLAB Function/7(Y7) -> Unit Delay4/1
  Data Type Conversion6/1 -> [X7]
  [X8] -> MATLAB Function/9(X8)
  [X7] -> MATLAB Function/8(X7)
  [X6] -> MATLAB Function/7(X6)
  [X5] -> MATLAB Function/6(X5)
  Data Type Conversion5/1 -> [X6]
  Data Type Conversion4/1 -> [X5]
  MATLAB Function/5(Y5) -> Unit Delay5/1
  MATLAB Function/6(Y6) -> Unit Delay6/1
  Unit Delay5/1 -> Data Type Conversion4/1
  Unit Delay6/1 -> Data Type Conversion5/1
  [X4] -> MATLAB Function/5(X4)
  [X3] -> MATLAB Function/4(X3)
  [X2] -> MATLAB Function/3(X2)
  Unit Delay3/1 -> Data Type Conversion3/1
  Unit Delay2/1 -> Data Type Conversion2/1
  Unit Delay1/1 -> Data Type Conversion1/1
  MATLAB Function/4(Y4) -> Unit Delay3/1
  MATLAB Function/3(Y3) -> Unit Delay2/1
  MATLAB Function/2(Y2) -> Unit Delay1/1
  C/1 -> MATLAB Function/1(C)
  MATLAB Function/1(S) -> Data Type Conversion9/1
  LFM1/1 -> MATLAB Function/2(Min)
  Data Type Conversion1/1 -> [X2]
  Data Type Conversion2/1 -> [X3]
  Data Type Conversion3/1 -> [X4]
  Data Type Conversion9/1 -> S/1

== system tpm/TPM/TPMS/TPMS/Learn/AutoLocation/IDIdentify/Subsystem2/Enabled Subsystem2 ==
  C : Inport
  LFM1 : Inport  Port=2
  Enable : EnablePort
  Data Type Conversion{1..8} (8 alike) : DataTypeConversion  OutDataTypeStr=int16
  Data Type Conversion9 : DataTypeConversion  OutDataTypeStr=uint8
  MATLAB Function : MATLAB Function  TreatAsAtomicUnit=on
  Unit Delay{1..8} (8 alike) : UnitDelay  SampleTime=-1  HasFrameUpgradeWarning=on
  S : Outport
  wires:
  Data Type Conversion3/1 -> [X4]
  Data Type Conversion2/1 -> [X3]
  Data Type Conversion1/1 -> [X2]
  LFM1/1 -> MATLAB Function/2(Min)
  MATLAB Function/1(S) -> Data Type Conversion9/1
  C/1 -> MATLAB Function/1(C)
  MATLAB Function/2(Y2) -> Unit Delay1/1
  MATLAB Function/3(Y3) -> Unit Delay2/1
  MATLAB Function/4(Y4) -> Unit Delay3/1
  Unit Delay1/1 -> Data Type Conversion1/1
  Unit Delay2/1 -> Data Type Conversion2/1
  Unit Delay3/1 -> Data Type Conversion3/1
  [X2] -> MATLAB Function/3(X2)
  [X3] -> MATLAB Function/4(X3)
  [X4] -> MATLAB Function/5(X4)
  Unit Delay6/1 -> Data Type Conversion5/1
  Unit Delay5/1 -> Data Type Conversion4/1
  MATLAB Function/6(Y6) -> Unit Delay6/1
  MATLAB Function/5(Y5) -> Unit Delay5/1
  Data Type Conversion4/1 -> [X5]
  Data Type Conversion5/1 -> [X6]
  [X5] -> MATLAB Function/6(X5)
  [X6] -> MATLAB Function/7(X6)
  [X7] -> MATLAB Function/8(X7)
  [X8] -> MATLAB Function/9(X8)
  Data Type Conversion6/1 -> [X7]
  MATLAB Function/7(Y7) -> Unit Delay4/1
  Unit Delay4/1 -> Data Type Conversion6/1
  Unit Delay7/1 -> Data Type Conversion7/1
  Data Type Conversion7/1 -> [X8]
  MATLAB Function/8(Y8) -> Unit Delay7/1
  MATLAB Function/9(Y9) -> Unit Delay8/1
  Data Type Conversion8/1 -> [X9]
  Unit Delay8/1 -> Data Type Conversion8/1
  [X9] -> MATLAB Function/10(X9)
  Data Type Conversion9/1 -> S/1

== system tpm/TPM/TPMS/TPMS/Learn/AutoLocation/IDIdentify/Subsystem2/Enabled Subsystem3 ==
  C : Inport
  LFM1 : Inport  Port=2
  Enable : EnablePort
  Data Type Conversion{1..8} (8 alike) : DataTypeConversion  OutDataTypeStr=int16
  Data Type Conversion9 : DataTypeConversion  OutDataTypeStr=uint8
  MATLAB Function : MATLAB Function  TreatAsAtomicUnit=on
  Unit Delay{1..8} (8 alike) : UnitDelay  SampleTime=-1  HasFrameUpgradeWarning=on
  S : Outport
  wires:
  [X9] -> MATLAB Function/10(X9)
  Unit Delay8/1 -> Data Type Conversion8/1
  Data Type Conversion8/1 -> [X9]
  MATLAB Function/9(Y9) -> Unit Delay8/1
  MATLAB Function/8(Y8) -> Unit Delay7/1
  Data Type Conversion7/1 -> [X8]
  Unit Delay7/1 -> Data Type Conversion7/1
  Unit Delay4/1 -> Data Type Conversion6/1
  MATLAB Function/7(Y7) -> Unit Delay4/1
  Data Type Conversion6/1 -> [X7]
  [X8] -> MATLAB Function/9(X8)
  [X7] -> MATLAB Function/8(X7)
  [X6] -> MATLAB Function/7(X6)
  [X5] -> MATLAB Function/6(X5)
  Data Type Conversion5/1 -> [X6]
  Data Type Conversion4/1 -> [X5]
  MATLAB Function/5(Y5) -> Unit Delay5/1
  MATLAB Function/6(Y6) -> Unit Delay6/1
  Unit Delay5/1 -> Data Type Conversion4/1
  Unit Delay6/1 -> Data Type Conversion5/1
  [X4] -> MATLAB Function/5(X4)
  [X3] -> MATLAB Function/4(X3)
  [X2] -> MATLAB Function/3(X2)
  Unit Delay3/1 -> Data Type Conversion3/1
  Unit Delay2/1 -> Data Type Conversion2/1
  Unit Delay1/1 -> Data Type Conversion1/1
  MATLAB Function/4(Y4) -> Unit Delay3/1
  MATLAB Function/3(Y3) -> Unit Delay2/1
  MATLAB Function/2(Y2) -> Unit Delay1/1
  C/1 -> MATLAB Function/1(C)
  MATLAB Function/1(S) -> Data Type Conversion9/1
  LFM1/1 -> MATLAB Function/2(Min)
  Data Type Conversion1/1 -> [X2]
  Data Type Conversion2/1 -> [X3]
  Data Type Conversion3/1 -> [X4]
  Data Type Conversion9/1 -> S/1

== system tpm/TPM/TPMS/TPMS/Learn/AutoLocation/IDIdentify/Subsystem2/Enabled Subsystem5 ==
  C : Inport
  LFM1 : Inport  Port=2
  Enable : EnablePort
  Data Type Conversion{1..8} (8 alike) : DataTypeConversion  OutDataTypeStr=int16
  Data Type Conversion9 : DataTypeConversion  OutDataTypeStr=uint8
  MATLAB Function : MATLAB Function  TreatAsAtomicUnit=on
  Unit Delay{1..8} (8 alike) : UnitDelay  SampleTime=-1  HasFrameUpgradeWarning=on
  S : Outport
  wires:
  Data Type Conversion3/1 -> [X4]
  Data Type Conversion2/1 -> [X3]
  Data Type Conversion1/1 -> [X2]
  LFM1/1 -> MATLAB Function/2(Min)
  MATLAB Function/1(S) -> Data Type Conversion9/1
  C/1 -> MATLAB Function/1(C)
  MATLAB Function/2(Y2) -> Unit Delay1/1
  MATLAB Function/3(Y3) -> Unit Delay2/1
  MATLAB Function/4(Y4) -> Unit Delay3/1
  Unit Delay1/1 -> Data Type Conversion1/1
  Unit Delay2/1 -> Data Type Conversion2/1
  Unit Delay3/1 -> Data Type Conversion3/1
  [X2] -> MATLAB Function/3(X2)
  [X3] -> MATLAB Function/4(X3)
  [X4] -> MATLAB Function/5(X4)
  Unit Delay6/1 -> Data Type Conversion5/1
  Unit Delay5/1 -> Data Type Conversion4/1
  MATLAB Function/6(Y6) -> Unit Delay6/1
  MATLAB Function/5(Y5) -> Unit Delay5/1
  Data Type Conversion4/1 -> [X5]
  Data Type Conversion5/1 -> [X6]
  [X5] -> MATLAB Function/6(X5)
  [X6] -> MATLAB Function/7(X6)
  [X7] -> MATLAB Function/8(X7)
  [X8] -> MATLAB Function/9(X8)
  Data Type Conversion6/1 -> [X7]
  MATLAB Function/7(Y7) -> Unit Delay4/1
  Unit Delay4/1 -> Data Type Conversion6/1
  Unit Delay7/1 -> Data Type Conversion7/1
  Data Type Conversion7/1 -> [X8]
  MATLAB Function/8(Y8) -> Unit Delay7/1
  MATLAB Function/9(Y9) -> Unit Delay8/1
  Data Type Conversion8/1 -> [X9]
  Unit Delay8/1 -> Data Type Conversion8/1
  [X9] -> MATLAB Function/10(X9)
  Data Type Conversion9/1 -> S/1

== system tpm/TPM/TPMS/TPMS/Learn/AutoLocation/IDIdentify/Subsystem3/Enabled Subsystem1 ==
  C : Inport
  LFM1 : Inport  Port=2
  Enable : EnablePort
  Data Type Conversion{1..8} (8 alike) : DataTypeConversion  OutDataTypeStr=int16
  Data Type Conversion9 : DataTypeConversion  OutDataTypeStr=uint8
  MATLAB Function : MATLAB Function  TreatAsAtomicUnit=on
  Unit Delay{1..8} (8 alike) : UnitDelay  SampleTime=-1  HasFrameUpgradeWarning=on
  S : Outport
  wires:
  Data Type Conversion9/1 -> S/1
  Data Type Conversion3/1 -> [X4]
  Data Type Conversion2/1 -> [X3]
  Data Type Conversion1/1 -> [X2]
  LFM1/1 -> MATLAB Function/2(Min)
  MATLAB Function/1(S) -> Data Type Conversion9/1
  C/1 -> MATLAB Function/1(C)
  MATLAB Function/2(Y2) -> Unit Delay1/1
  MATLAB Function/3(Y3) -> Unit Delay2/1
  MATLAB Function/4(Y4) -> Unit Delay3/1
  Unit Delay1/1 -> Data Type Conversion1/1
  Unit Delay2/1 -> Data Type Conversion2/1
  Unit Delay3/1 -> Data Type Conversion3/1
  [X2] -> MATLAB Function/3(X2)
  [X3] -> MATLAB Function/4(X3)
  [X4] -> MATLAB Function/5(X4)
  Unit Delay6/1 -> Data Type Conversion5/1
  Unit Delay5/1 -> Data Type Conversion4/1
  MATLAB Function/6(Y6) -> Unit Delay6/1
  MATLAB Function/5(Y5) -> Unit Delay5/1
  Data Type Conversion4/1 -> [X5]
  Data Type Conversion5/1 -> [X6]
  [X5] -> MATLAB Function/6(X5)
  [X6] -> MATLAB Function/7(X6)
  [X7] -> MATLAB Function/8(X7)
  [X8] -> MATLAB Function/9(X8)
  Data Type Conversion6/1 -> [X7]
  MATLAB Function/7(Y7) -> Unit Delay4/1
  Unit Delay4/1 -> Data Type Conversion6/1
  Unit Delay7/1 -> Data Type Conversion7/1
  Data Type Conversion7/1 -> [X8]
  MATLAB Function/8(Y8) -> Unit Delay7/1
  MATLAB Function/9(Y9) -> Unit Delay8/1
  Data Type Conversion8/1 -> [X9]
  Unit Delay8/1 -> Data Type Conversion8/1
  [X9] -> MATLAB Function/10(X9)

== system tpm/TPM/TPMS/TPMS/Learn/AutoLocation/IDIdentify/Subsystem3/Enabled Subsystem2 ==
  C : Inport
  LFM1 : Inport  Port=2
  Enable : EnablePort
  Data Type Conversion{1..8} (8 alike) : DataTypeConversion  OutDataTypeStr=int16
  Data Type Conversion9 : DataTypeConversion  OutDataTypeStr=uint8
  MATLAB Function : MATLAB Function  TreatAsAtomicUnit=on
  Unit Delay{1..8} (8 alike) : UnitDelay  SampleTime=-1  HasFrameUpgradeWarning=on
  S : Outport
  wires:
  Data Type Conversion9/1 -> S/1
  [X9] -> MATLAB Function/10(X9)
  Unit Delay8/1 -> Data Type Conversion8/1
  Data Type Conversion8/1 -> [X9]
  MATLAB Function/9(Y9) -> Unit Delay8/1
  MATLAB Function/8(Y8) -> Unit Delay7/1
  Data Type Conversion7/1 -> [X8]
  Unit Delay7/1 -> Data Type Conversion7/1
  Unit Delay4/1 -> Data Type Conversion6/1
  MATLAB Function/7(Y7) -> Unit Delay4/1
  Data Type Conversion6/1 -> [X7]
  [X8] -> MATLAB Function/9(X8)
  [X7] -> MATLAB Function/8(X7)
  [X6] -> MATLAB Function/7(X6)
  [X5] -> MATLAB Function/6(X5)
  Data Type Conversion5/1 -> [X6]
  Data Type Conversion4/1 -> [X5]
  MATLAB Function/5(Y5) -> Unit Delay5/1
  MATLAB Function/6(Y6) -> Unit Delay6/1
  Unit Delay5/1 -> Data Type Conversion4/1
  Unit Delay6/1 -> Data Type Conversion5/1
  [X4] -> MATLAB Function/5(X4)
  [X3] -> MATLAB Function/4(X3)
  [X2] -> MATLAB Function/3(X2)
  Unit Delay3/1 -> Data Type Conversion3/1
  Unit Delay2/1 -> Data Type Conversion2/1
  Unit Delay1/1 -> Data Type Conversion1/1
  MATLAB Function/4(Y4) -> Unit Delay3/1
  MATLAB Function/3(Y3) -> Unit Delay2/1
  MATLAB Function/2(Y2) -> Unit Delay1/1
  C/1 -> MATLAB Function/1(C)
  MATLAB Function/1(S) -> Data Type Conversion9/1
  LFM1/1 -> MATLAB Function/2(Min)
  Data Type Conversion1/1 -> [X2]
  Data Type Conversion2/1 -> [X3]
  Data Type Conversion3/1 -> [X4]

== system tpm/TPM/TPMS/TPMS/Learn/AutoLocation/IDIdentify/Subsystem3/Enabled Subsystem3 ==
  C : Inport
  LFM1 : Inport  Port=2
  Enable : EnablePort
  Data Type Conversion{1..8} (8 alike) : DataTypeConversion  OutDataTypeStr=int16
  Data Type Conversion9 : DataTypeConversion  OutDataTypeStr=uint8
  MATLAB Function : MATLAB Function  TreatAsAtomicUnit=on
  Unit Delay{1..8} (8 alike) : UnitDelay  SampleTime=-1  HasFrameUpgradeWarning=on
  S : Outport
  wires:
  Data Type Conversion9/1 -> S/1
  Data Type Conversion3/1 -> [X4]
  Data Type Conversion2/1 -> [X3]
  Data Type Conversion1/1 -> [X2]
  LFM1/1 -> MATLAB Function/2(Min)
  MATLAB Function/1(S) -> Data Type Conversion9/1
  C/1 -> MATLAB Function/1(C)
  MATLAB Function/2(Y2) -> Unit Delay1/1
  MATLAB Function/3(Y3) -> Unit Delay2/1
  MATLAB Function/4(Y4) -> Unit Delay3/1
  Unit Delay1/1 -> Data Type Conversion1/1
  Unit Delay2/1 -> Data Type Conversion2/1
  Unit Delay3/1 -> Data Type Conversion3/1
  [X2] -> MATLAB Function/3(X2)
  [X3] -> MATLAB Function/4(X3)
  [X4] -> MATLAB Function/5(X4)
  Unit Delay6/1 -> Data Type Conversion5/1
  Unit Delay5/1 -> Data Type Conversion4/1
  MATLAB Function/6(Y6) -> Unit Delay6/1
  MATLAB Function/5(Y5) -> Unit Delay5/1
  Data Type Conversion4/1 -> [X5]
  Data Type Conversion5/1 -> [X6]
  [X5] -> MATLAB Function/6(X5)
  [X6] -> MATLAB Function/7(X6)
  [X7] -> MATLAB Function/8(X7)
  [X8] -> MATLAB Function/9(X8)
  Data Type Conversion6/1 -> [X7]
  MATLAB Function/7(Y7) -> Unit Delay4/1
  Unit Delay4/1 -> Data Type Conversion6/1
  Unit Delay7/1 -> Data Type Conversion7/1
  Data Type Conversion7/1 -> [X8]
  MATLAB Function/8(Y8) -> Unit Delay7/1
  MATLAB Function/9(Y9) -> Unit Delay8/1
  Data Type Conversion8/1 -> [X9]
  Unit Delay8/1 -> Data Type Conversion8/1
  [X9] -> MATLAB Function/10(X9)

== system tpm/TPM/TPMS/TPMS/Learn/AutoLocation/IDIdentify/Subsystem3/Enabled Subsystem5 ==
  C : Inport
  LFM1 : Inport  Port=2
  Enable : EnablePort
  Data Type Conversion{1..8} (8 alike) : DataTypeConversion  OutDataTypeStr=int16
  Data Type Conversion9 : DataTypeConversion  OutDataTypeStr=uint8
  MATLAB Function : MATLAB Function  TreatAsAtomicUnit=on
  Unit Delay{1..8} (8 alike) : UnitDelay  SampleTime=-1  HasFrameUpgradeWarning=on
  S : Outport
  wires:
  Data Type Conversion9/1 -> S/1
  [X9] -> MATLAB Function/10(X9)
  Unit Delay8/1 -> Data Type Conversion8/1
  Data Type Conversion8/1 -> [X9]
  MATLAB Function/9(Y9) -> Unit Delay8/1
  MATLAB Function/8(Y8) -> Unit Delay7/1
  Data Type Conversion7/1 -> [X8]
  Unit Delay7/1 -> Data Type Conversion7/1
  Unit Delay4/1 -> Data Type Conversion6/1
  MATLAB Function/7(Y7) -> Unit Delay4/1
  Data Type Conversion6/1 -> [X7]
  [X8] -> MATLAB Function/9(X8)
  [X7] -> MATLAB Function/8(X7)
  [X6] -> MATLAB Function/7(X6)
  [X5] -> MATLAB Function/6(X5)
  Data Type Conversion5/1 -> [X6]
  Data Type Conversion4/1 -> [X5]
  MATLAB Function/5(Y5) -> Unit Delay5/1
  MATLAB Function/6(Y6) -> Unit Delay6/1
  Unit Delay5/1 -> Data Type Conversion4/1
  Unit Delay6/1 -> Data Type Conversion5/1
  [X4] -> MATLAB Function/5(X4)
  [X3] -> MATLAB Function/4(X3)
  [X2] -> MATLAB Function/3(X2)
  Unit Delay3/1 -> Data Type Conversion3/1
  Unit Delay2/1 -> Data Type Conversion2/1
  Unit Delay1/1 -> Data Type Conversion1/1
  MATLAB Function/4(Y4) -> Unit Delay3/1
  MATLAB Function/3(Y3) -> Unit Delay2/1
  MATLAB Function/2(Y2) -> Unit Delay1/1
  C/1 -> MATLAB Function/1(C)
  MATLAB Function/1(S) -> Data Type Conversion9/1
  LFM1/1 -> MATLAB Function/2(Min)
  Data Type Conversion1/1 -> [X2]
  Data Type Conversion2/1 -> [X3]
  Data Type Conversion3/1 -> [X4]
